simulink model "Copy_of_nonlinear_model1"  (R2021b)
settings: Solver=FixedStepAuto  StartTime=0.0  StopTime=RunTime  FixedStep=time_step  RelTol=1e-3
values from neighbouring files (symbols this model uses):
  init_theta_1 = pi    (= 3.14159265359)    [compare_ourmodel_with_others.m]    (also in step2_whitebox_beam.m = theta_1(1); step2_whitebox_pend.m)
  init_theta_2 = 0    [compare_ourmodel_with_others.m]    (also in step2_whitebox_beam.m = theta_1(2); step2_whitebox_pend.m = -1.57079632679)
  params_hat = params    [costfun.m]    (also in step2_whitebox_beam.m = params_init)
settings Model: Creator=97083  LastModifiedBy=lyitingli
settings DataIOCC: ExternalInput=[u]
settings DebuggingCC: UnconnectedInputMsg=none  UnconnectedOutputMsg=none  UnconnectedLineMsg=none  UnderSpecifiedDimensionMsg=warning
settings ModelReferenceCC: EnableRefExpFcnMdlSchedulingChecks=off
settings RTWCC: DLArmComputeVersion=20.02.1

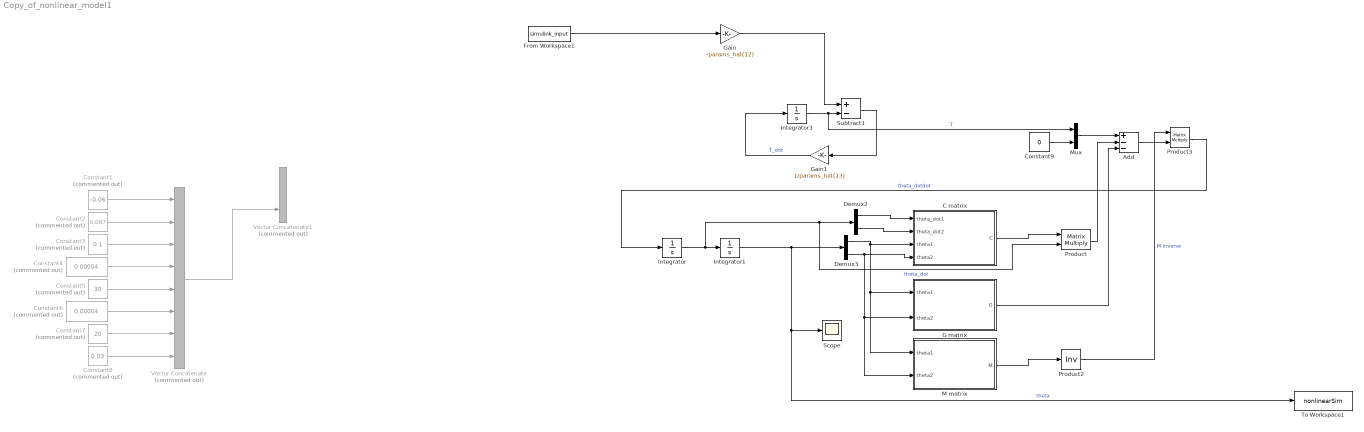
== system Copy_of_nonlinear_model1 ==
  Add : Sum  Inputs=+--
  C matrix : MATLAB Function  TreatAsAtomicUnit=on
  Constant1 : Constant  Commented=on  Value=-0.06
  Constant2 : Constant  Commented=on  Value=0.087
  Constant3 : Constant  Commented=on  Value=0.1
  Constant4 : Constant  Commented=on  Value=0.00004
  Constant5 : Constant  Commented=on  Value=30
  Constant6 : Constant  Commented=on  Value=0.00004
  Constant7 : Constant  Commented=on  Value=20
  Constant8 : Constant  Commented=on  Value=0.03
  Constant9 : Constant  Value=0
  Demux2 : Demux  Outputs=2
  Demux3 : Demux  Outputs=2
  From Workspace1 : FromWorkspace  SampleTime=-1
  G matrix : MATLAB Function  TreatAsAtomicUnit=on
  Gain : Gain  Gain=-params_hat(12)
  Gain1 : Gain  Gain=1/params_hat(13)
  Integrator : Integrator
  Integrator1 : Integrator  InitialCondition=[init_theta_1, init_theta_2]
  Integrator3 : Integrator
  M matrix : MATLAB Function  TreatAsAtomicUnit=on
  Mux : Mux  Inputs=2
  Product : Product  Inputs=**  Multiplication=Matrix(*)
  Product2 : Product  Inputs=/  Multiplication=Matrix(*)
  Product3 : Product  Inputs=**  Multiplication=Matrix(*)
  Scope : Scope
  Subtract1 : Sum  Inputs=+-
  To Workspace1 : ToWorkspace  VariableName=nonlinearSim  SampleTime=0.001
  Vector Concatenate : Concatenate  Commented=on  NumInputs=8
  Vector Concatenate1 : Concatenate  Commented=on
  wires:
  Constant1/1 -> Vector Concatenate/1
  Constant2/1 -> Vector Concatenate/2
  Constant3/1 -> Vector Concatenate/3
  Constant4/1 -> Vector Concatenate/4
  Constant5/1 -> Vector Concatenate/5
  Constant6/1 -> Vector Concatenate/6
  Constant7/1 -> Vector Concatenate/7
  Constant8/1 -> Vector Concatenate/8
  Vector Concatenate/1 -> Vector Concatenate1/2
  G matrix/1(G) -> Add/3
  From Workspace1/1 -> Gain/1
  Product/1 -> Add/2
  Subtract1/1 -> Gain1/1
  Add/1 -> Product3/2
  Demux2/1 -> C matrix/1(theta_dot1)
  Constant9/1 -> Mux/2
  Integrator3/1 -> Mux/1, Subtract1/2  "T"
  Gain1/1 -> Integrator3/1  "T_dot"
  Demux3/1 -> M matrix/1(theta1), G matrix/1(theta1), C matrix/3(theta1)
  Product2/1 -> Product3/1  "M inverse"
  Product3/1 -> Integrator/1  "theta_dotdot"
  Gain/1 -> Subtract1/1
  Demux3/2 -> M matrix/2(theta2), G matrix/2(theta2), C matrix/4(theta2)
  M matrix/1(M) -> Product2/1
  Demux2/2 -> C matrix/2(theta_dot2)
  Integrator1/1 -> Demux3/1, To Workspace1/1, Scope/1  "theta"
  Mux/1 -> Add/1
  C matrix/1(C) -> Product/1
  Integrator/1 -> Product/2, Demux2/1, Integrator1/1  "theta_dot"

== matlab function Copy_of_nonlinear_model1/C matrix ==
  data: theta_dot1 input; theta_dot2 input; theta1 input; theta2 input; C output; params_hat parameter
function C = C(theta_dot1, theta_dot2, theta1, theta2, params_hat)
l_1 = params_hat(2);
m_2 = params_hat(5);
P3 = m_2 * l_1 * params_hat(7);

C00 = params_hat(10) - P3 * theta_dot2 * sin(theta2);
C01 = -P3 * (theta_dot1 + theta_dot2) * sin(theta2);
C10 = P3 * theta_dot1 * sin(theta2);
C11 = params_hat(11);

C = [C00 C01; C10 C11];

== matlab function Copy_of_nonlinear_model1/G matrix ==
  data: theta1 input; theta2 input; G output; params_hat parameter
function G = G(theta1, theta2, params_hat)
g = params_hat(1);
l_1 = params_hat(2);
m_1 = params_hat(4);
m_2 = params_hat(5);

c_1_0 = params_hat(6);
c_2_0 = params_hat(7);

g1 = (m_1 * c_1_0 + m_2 * l_1) * g;
g2 = m_2 * c_2_0 * g;

G00 = -g1 * sin(theta1) - g2 * sin(theta1 + theta2);
G01 = -g2 * sin(theta1 + theta2);

G = [G00 G01];

== matlab function Copy_of_nonlinear_model1/M matrix ==
  data: theta1 input; theta2 input; M output; params_hat parameter
function M = M(theta1, theta2, params_hat)
g = params_hat(1);
l_1 = params_hat(2);
m_1 = params_hat(4);
m_2 = params_hat(5);

c_1_0 = params_hat(6);
c_2_0 = params_hat(7);
I_1_0 = params_hat(8);
I_2_0 = params_hat(9);
P1 = m_1 * c_1_0 * c_1_0 + m_2 * l_1 * l_1 + I_1_0;
P2 = m_2 * c_2_0 * c_2_0 + I_2_0;
P3 = m_2 * l_1 * c_2_0;


M00 = P1 + P2 + 2 * P3 * cos(theta2);
M01 = P2 + P3 * cos(theta2);
M10 = M01;
M11 = P2;

M = [M00 M01; M10 M11];
